simulink model "Vehicle_HIL_plant"  (R2022b)
settings: Solver=VariableStepAuto  StartTime=0.0  StopTime=inf  RelTol=1e-3
undefined symbols (not defined in the file): canChannel, MI_STATUSES
libraries: canmsglib x12, canlib x5, dspstat3 x4, simulink x2, realtime_pacer_lib x1, battery_monitor_lib x1, driver_interface_lib x1, governor_lib x1, motor_interface_lib x1, simp_vd_lib x1
settings Model: Creator=LinF  LastModifiedBy=LinF

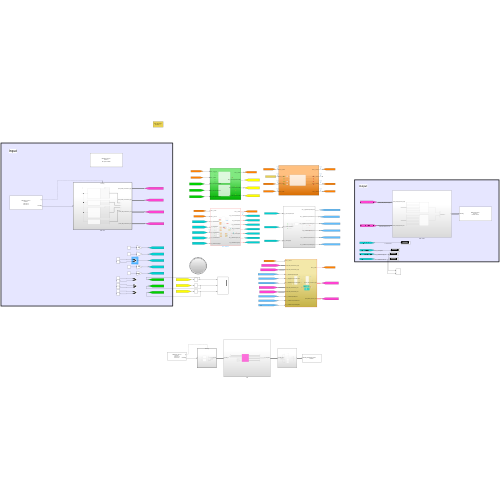
[thumbnail: Simulink's stored preview of the top-level diagram]
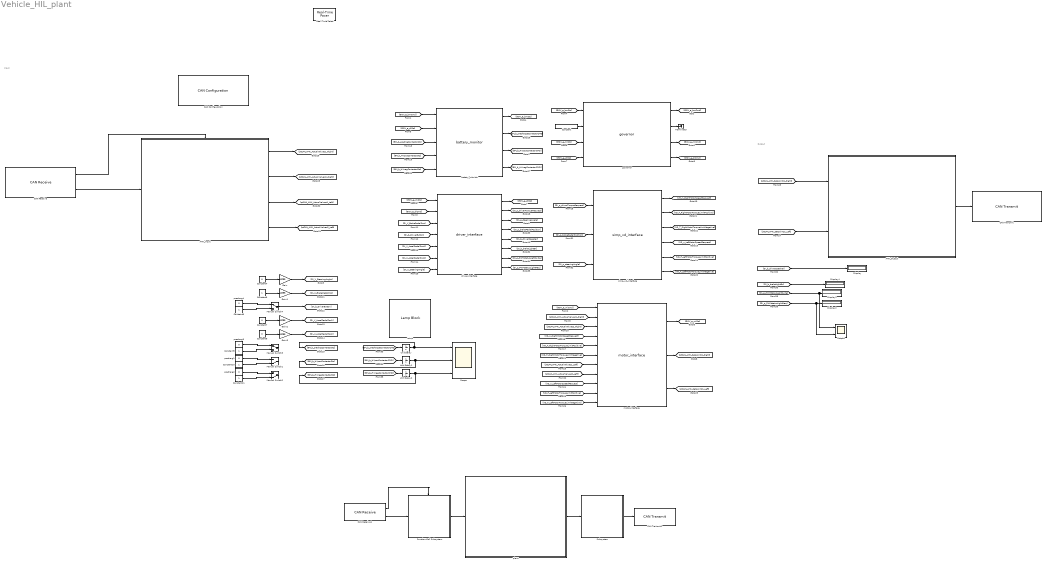
== system Vehicle_HIL_plant ==
  note: Input
  note: Output
  AMK_Input : Subsystem  TreatAsAtomicUnit=on
  AMK_Output : Subsystem
  CAN Configuration : canlib/CAN Configuration  BlockHandle=174.0005  Device=MathWorks Virtual 1 (Channel 1)  DeviceMenu=MathWorks Virtual 1 (Channel 1)  ObjConstructor=canChannel('MathWorks', 'Virtual 1', 1)  BusSpeed=500000  EnableBitParameters=off  AckMode=Normal
  CAN Receive : canlib/CAN Receive  BlockHandle=175.0005  Device=MathWorks Virtual 1 (Channel 1)  DeviceMenu=MathWorks Virtual 1 (Channel 1)  ObjConstructor=canChannel('MathWorks', 'Virtual 1', 1)  EnableStandardIDsFilter=off  StdIDsCombo=Allow all  StandardIDs=0  EnableExtendedIDsFilter=off  ExtIDsCombo=Allow all  ExtendedIDs=0  SampleTime=0.005  MsgsPerTimestep=all  InternalFilterUpdateStatus=on  BusOutput=off
  CAN Receive1 : canlib/CAN Receive  BlockHandle=178.0005  Device=MathWorks Virtual 1 (Channel 1)  DeviceMenu=MathWorks Virtual 1 (Channel 1)  ObjConstructor=canChannel('MathWorks', 'Virtual 1', 1)  EnableStandardIDsFilter=off  StdIDsCombo=Allow all  StandardIDs=0  EnableExtendedIDsFilter=off  ExtIDsCombo=Allow all  ExtendedIDs=0  SampleTime=0.005  MsgsPerTimestep=all  InternalFilterUpdateStatus=on  BusOutput=off
  CAN Transmit : canlib/CAN Transmit  BlockHandle=181.0005  Device=MathWorks Virtual 1 (Channel 1)  DeviceMenu=MathWorks Virtual 1 (Channel 1)  ObjConstructor=canChannel('MathWorks', 'Virtual 1', 1)  EnableEventTransmit=off  EnablePeriodicTransmit=on  MessagePeriod=0.005
  CAN Transmit1 : canlib/CAN Transmit  BlockHandle=183.0005  Device=MathWorks Virtual 1 (Channel 1)  DeviceMenu=MathWorks Virtual 1 (Channel 1)  ObjConstructor=canChannel('MathWorks', 'Virtual 1', 1)  EnableEventTransmit=off  EnablePeriodicTransmit=off  MessagePeriod=1.000
  Constant : Constant  Value=MI_STATUSES.STS_INIT  OutDataTypeStr=Enum: MI_STATUSES
  Constant{5..6,9..11} (5 alike) : Constant
  Constant4 : Constant  Value=0
  Constant7 : Constant  Value=0
  Constant8 : Constant  Value=0
  Display{,1..2,4} (4 alike) : Display
  Function-Call Subsystem : Subsystem  TreatAsAtomicUnit=on
  Gain{,1..3} (4 alike) : Gain  Gain=4095
  Lamp : LampBlock  LabelPosition=Hide
  Manual Switch1 : ManualSwitch  CurrentSetting=0
  Manual Switch2 : ManualSwitch  CurrentSetting=0
  Manual Switch3 : ManualSwitch
  Manual Switch4 : ManualSwitch
  Real-Time Pacer : realtime_pacer_lib/Real-Time Pacer  simTimePerRealTime=1
  Scope : Scope  NumInputPorts=3
  Scope1 : Scope  NumInputPorts=2
  Subsystem : Subsystem
  Terminator : Terminator
  Unit Delay : UnitDelay  SampleTime=-1  HasFrameUpgradeWarning=on
  Unit Delay1 : UnitDelay  SampleTime=-1  HasFrameUpgradeWarning=on
  Unit Delay2 : UnitDelay  SampleTime=-1  HasFrameUpgradeWarning=on
  battery_monitor : battery_monitor_lib/battery_monitor  SystemSampleTime=-1  VariantActivationTime=update diagram  Latency=0  AutoFrameSizeCalculation=off
  driver_interface : driver_interface_lib/driver_interface  SystemSampleTime=-1  VariantActivationTime=update diagram  Latency=0  AutoFrameSizeCalculation=off
  governor : governor_lib/governor  SystemSampleTime=-1  VariantActivationTime=update diagram  Latency=0  AutoFrameSizeCalculation=off
  motor_interface : motor_interface_lib/motor_interface  SystemSampleTime=-1  VariantActivationTime=update diagram  Latency=0  AutoFrameSizeCalculation=off
  plant : Subsystem
      settings: LibrarySourceBlock=plant_lib/plant
  precharg{1..4} (4 alike) : Constant  Value=0
  simp_vd_interface : simp_vd_lib/simp_vd_interface  SystemSampleTime=-1  VariantActivationTime=update diagram  Latency=0  AutoFrameSizeCalculation=off
  wires:
  Function-Call Subsystem/1(pt_CAN_IN) -> plant/1(pt_CAN_IN)
  CAN Receive1/2 -> Function-Call Subsystem/1(In1)
  CAN Receive1/1 -> Function-Call Subsystem/Trigger
  plant/1(pt_CAN_OUT) -> Subsystem/1(pt_CAN_OUT)
  Subsystem/1(Out1) -> CAN Transmit1/1
  Gain3/1 -> [DI_V_AccelPedalPos2]
  [DI_b_driverSpeaker] -> Display/1  "DI_b_driverSpeaker"
  Constant4/1 -> Gain/1
  Gain2/1 -> [DI_V_AccelPedalPos1]
  Manual Switch4/1 -> [DI_b_DriverButton]
  Gain1/1 -> [DI_V_BrakePedalPos]
  motor_interface/1 -> [GOV_e_miSts]
  [ptCAN_AMK_Setpoints1_Right] -> AMK_Output/1(ptCAN_AMK_Setpoints1_Right)  "ptCAN_AMK_Setpoints1_Right"
  Constant5/1 -> Gain1/1
  [VD_T_RightMotorTorqueLimitPositive] -> motor_interface/5
  [GOV_e_bmSts] -> governor/1
  AMK_Input/2(ptCAN_AMK_ActualValues2_Right) -> [ptCAN_AMK_ActualValues2_Right]
  CAN Receive/1 -> AMK_Input/Trigger
  AMK_Output/1(Out1) -> CAN Transmit/1
  AMK_Input/4(ptCAN_AMK_ActualValues2_Left) -> [ptCAN_AMK_ActualValues2_Left]
  AMK_Input/3(ptCAN_AMK_ActualValues1_Left) -> [ptCAN_AMK_ActualValues1_Left]
  CAN Receive/2 -> AMK_Input/1(In1)
  motor_interface/3 -> [ptCAN_AMK_Setpoints1_Left]
  governor/1 -> [GOV_e_bmCmd]
  governor/2 -> Terminator/1
  governor/4 -> [GOV_e_diCmd]
  motor_interface/2 -> [ptCAN_AMK_Setpoints1_Right]
  [GOV_e_diSts] -> governor/4
  [VD_T_LeftMotorTorqueLimitPositive] -> motor_interface/10
  [VD_T_RightMotorTorqueLimitNegative] -> motor_interface/6
  [VD_n_RightMotorSpeedRequest] -> motor_interface/4
  [GOV_e_miCmd] -> motor_interface/1
  [VD_T_LeftMotorTorqueLimitNegative] -> motor_interface/11
  [VD_n_LeftMotorSpeedRequest] -> motor_interface/9
  AMK_Input/1(ptCAN_AMK_ActualValues1_Right) -> [ptCAN_AMK_ActualValues1_Right]
  [ptCAN_AMK_ActualValues2_Left] -> motor_interface/8
  Constant/1 -> governor/2
  governor/3 -> [GOV_e_miCmd]
  [ptCAN_AMK_ActualValues1_Right] -> motor_interface/2
  [ptCAN_AMK_ActualValues2_Right] -> motor_interface/3
  [ptCAN_AMK_ActualValues1_Left] -> motor_interface/7
  [ptCAN_AMK_Setpoints1_Left] -> AMK_Output/2(ptCAN_AMK_Setpoints1_Left)  "ptCAN_AMK_Setpoints1_Left"
  Gain/1 -> [DI_V_SteeringAngle]
  Constant8/1 -> Gain3/1
  [GOV_e_miSts] -> governor/3
  Constant7/1 -> Gain2/1
  Constant10/1 -> Manual Switch1/2
  precharg1/1 -> Manual Switch1/1
  [BM_b_HVposContactorCMD] -> Unit Delay1/1
  precharg2/1 -> Manual Switch2/1
  Constant11/1 -> Manual Switch2/2
  [BM_b_HVnegContactorCMD] -> Unit Delay2/1
  precharg3/1 -> Manual Switch3/1
  Constant9/1 -> Manual Switch3/2
  [BM_b_prechargeContactorCMD] -> Unit Delay/1
  precharg4/1 -> Manual Switch4/1
  Constant6/1 -> Manual Switch4/2
  [BM_b_HVnegContactorSts] -> battery_monitor/5
  [GOV_e_bmCmd] -> battery_monitor/1
  battery_monitor/1 -> [GOV_e_bmSts]
  battery_monitor/2 -> [BM_b_prechargeContactorCMD]
  battery_monitor/3 -> [BM_b_HVposContactorCMD]
  [BM_b_prechrgContactorSts] -> battery_monitor/3
  battery_monitor/4 -> [BM_b_HVnegContactorCMD]
  [BM_b_HVposContactorSts] -> battery_monitor/4
  [GOV_e_diSts] -> battery_monitor/2
  Unit Delay/1 -> [BM_b_prechrgContactorSts], Scope/1
  Unit Delay1/1 -> [BM_b_HVposContactorSts], Scope/2
  Unit Delay2/1 -> [BM_b_HVnegContactorSts], Scope/3
  [DI_b_brakeLightEn] -> Display4/1  "DI_b_brakeLightEn"
  driver_interface/8 -> [DI_p_PWMstatusLightFreq]
  [GOV_e_miSts] -> driver_interface/1
  [GOV_e_diCmd] -> driver_interface/2
  [DI_V_AccelPedalPos1] -> driver_interface/5
  [DI_V_AccelPedalPos2] -> driver_interface/6
  driver_interface/6 -> [DI_b_brakeLightEn]
  [DI_b_DriverButton] -> driver_interface/4
  [DI_V_BrakePedalPos] -> driver_interface/3
  driver_interface/2 -> [DI_p_driverTorqueRequest]
  driver_interface/5 -> [DI_b_driverSpeaker]
  driver_interface/1 -> [GOV_e_diSts]
  driver_interface/4 -> [DI_p_brakePedalPosition]
  [DI_V_SteeringAngle] -> driver_interface/7
  driver_interface/3 -> [DI_p_steeringAngle]
  driver_interface/7 -> [DI_p_PWMstatusLightCycle]
  [DI_p_PWMstatusLightFreq] -> Scope1/2, Display2/1  "DI_p_PWMstatusLightFreq"
  [DI_p_PWMstatusLightCycle] -> Scope1/1, Display1/1  "DI_p_PWMstatusLightCycle"
  simp_vd_interface/4 -> [VD_n_LeftMotorSpeedRequest]
  simp_vd_interface/2 -> [VD_T_RightMotorTorqueLimitPositive]
  [DI_p_driverTorqueRequest] -> simp_vd_interface/1
  simp_vd_interface/6 -> [VD_T_LeftMotorTorqueLimitNegative]
  simp_vd_interface/3 -> [VD_T_RightMotorTorqueLimitNegative]
  [DI_p_steeringAngle] -> simp_vd_interface/3
  [DI_p_brakePedalPosition] -> simp_vd_interface/2
  simp_vd_interface/5 -> [VD_T_LeftMotorTorqueLimitPositive]
  simp_vd_interface/1 -> [VD_n_RightMotorSpeedRequest]

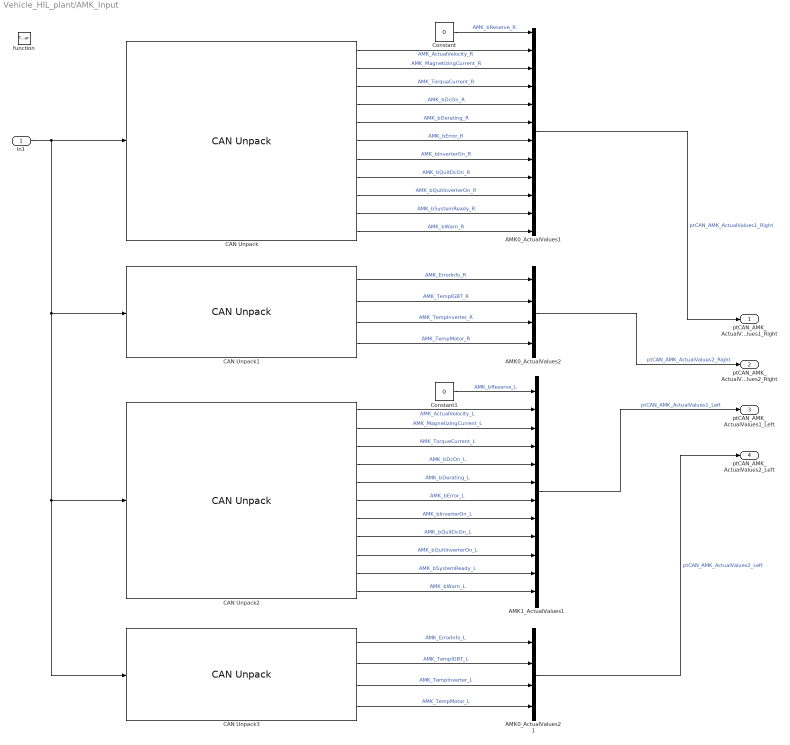
== system Vehicle_HIL_plant/AMK_Input ==
  In1 : Inport
  function : TriggerPort  TriggerType=function-call  VariantControl=(inherit)
  "AMK0_ActualValues1 " : BusCreator  Inputs=12
  "AMK0_ActualValues2 " : BusCreator  Inputs=4
  AMK0_ActualValues2 1 : BusCreator  Inputs=4
  AMK1_ActualValues1 : BusCreator  Inputs=12
  CAN Unpack : canmsglib/CAN Unpack  CANdbFile=C:\Users\LinF\Documents\MACFE\Embedded\CAN_Stuff\CAN_Databases\CAN_AMKInverter.dbc  MsgList=AMK1_ActualValues1  MsgName=AMK1_ActualValues1  MsgIDType=Standard (11-bit identifier)  MsgIdentifier=645  MsgLength=8  SignalInfo={'AMK_ActualVelocity','16','16','LE','signed','Standard','0','1','0','-Inf','Inf';'AMK_MagnetizingCurrent','48','16','LE','signed','Standard','0','1','0','-Inf','Inf';'AMK_TorqueCurrent','32','16','LE','signed','Standard','0','1','0','-Inf','Inf';'AMK_bDcOn','12','1','LE','unsigned','Standard','0','1','0','-Inf','Inf';'AMK_bDerating','15','1','LE','unsigned','Standard','0','1','0','-Inf','Inf';'AMK_bError','9','1','LE','unsigned','Standard','0','1','0','-Inf','Inf';'AMK_bInverterOn','14','1','LE','unsigned','Standard','0','1','0','-Inf','Inf';'AMK_bQuitDcOn','11','1','LE','unsigned','Standard','0','1','0','-Inf','Inf';'AMK_bQuitInverterOn','13','1','LE','unsigned','Standard','0','1','0','-Inf','Inf';'AMK_bSystemReady','8','1','LE','unsigned','Standard','0','1','0','-Inf','Inf';'AMK_bWarn','10','1','LE','unsigned','Standard','0','1','0','-Inf','Inf'}  IDPort=off  TimestampPort=off  ErrorPort=off  RemotePort=off  LengthPort=off  StatusPort=off  ApplyMinMax=off
      settings: LibrarySourceBlock=canlib/CAN Unpack  DataFormat=CANdb specified signals
  CAN Unpack1 : canmsglib/CAN Unpack  CANdbFile=C:\Users\LinF\Documents\MACFE\Embedded\CAN_Stuff\CAN_Databases\CAN_AMKInverter.dbc  MsgList=AMK1_ActualValues2  MsgName=AMK1_ActualValues2  MsgIDType=Standard (11-bit identifier)  MsgIdentifier=647  MsgLength=8  SignalInfo={'AMK_ErrorInfo','32','16','LE','unsigned','Standard','0','1','0','0','65535';'AMK_TempIGBT','48','16','LE','signed','Standard','0','0.1','0','-3276.8','3276.7';'AMK_TempInverter','16','16','LE','signed','Standard','0','0.1','0','-3276.8','3276.7';'AMK_TempMotor','0','16','LE','signed','Standard','0','0.1','0','-3276.8','3276.7'}  IDPort=off  TimestampPort=off  ErrorPort=off  RemotePort=off  LengthPort=off  StatusPort=off  ApplyMinMax=off
      settings: LibrarySourceBlock=canlib/CAN Unpack  DataFormat=CANdb specified signals
  CAN Unpack2 : canmsglib/CAN Unpack  CANdbFile=C:\Users\LinF\Documents\MACFE\Embedded\CAN_Stuff\CAN_Databases\CAN_AMKInverter.dbc  MsgList=AMK0_ActualValues1  MsgName=AMK0_ActualValues1  MsgIDType=Standard (11-bit identifier)  MsgIdentifier=644  MsgLength=8  SignalInfo={'AMK_ActualVelocity','16','16','LE','signed','Standard','0','1','0','-Inf','Inf';'AMK_MagnetizingCurrent','48','16','LE','signed','Standard','0','1','0','-Inf','Inf';'AMK_TorqueCurrent','32','16','LE','signed','Standard','0','1','0','-Inf','Inf';'AMK_bDcOn','12','1','LE','unsigned','Standard','0','1','0','-Inf','Inf';'AMK_bDerating','15','1','LE','unsigned','Standard','0','1','0','-Inf','Inf';'AMK_bError','9','1','LE','unsigned','Standard','0','1','0','-Inf','Inf';'AMK_bInverterOn','14','1','LE','unsigned','Standard','0','1','0','-Inf','Inf';'AMK_bQuitDcOn','11','1','LE','unsigned','Standard','0','1','0','-Inf','Inf';'AMK_bQuitInverterOn','13','1','LE','unsigned','Standard','0','1','0','-Inf','Inf';'AMK_bSystemReady','8','1','LE','unsigned','Standard','0','1','0','-Inf','Inf';'AMK_bWarn','10','1','LE','unsigned','Standard','0','1','0','-Inf','Inf'}  IDPort=off  TimestampPort=off  ErrorPort=off  RemotePort=off  LengthPort=off  StatusPort=off  ApplyMinMax=off
      settings: LibrarySourceBlock=canlib/CAN Unpack  DataFormat=CANdb specified signals
  CAN Unpack3 : canmsglib/CAN Unpack  CANdbFile=C:\Users\LinF\Documents\MACFE\Embedded\CAN_Stuff\CAN_Databases\CAN_AMKInverter.dbc  MsgList=AMK0_ActualValues2  MsgName=AMK0_ActualValues2  MsgIDType=Standard (11-bit identifier)  MsgIdentifier=646  MsgLength=8  SignalInfo={'AMK_ErrorInfo','32','16','LE','unsigned','Standard','0','1','0','0','65535';'AMK_TempIGBT','48','16','LE','signed','Standard','0','0.1','0','-3276.8','3276.7';'AMK_TempInverter','16','16','LE','signed','Standard','0','0.1','0','-3276.8','3276.7';'AMK_TempMotor','0','16','LE','signed','Standard','0','0.1','0','-3276.8','3276.7'}  IDPort=off  TimestampPort=off  ErrorPort=off  RemotePort=off  LengthPort=off  StatusPort=off  ApplyMinMax=off
      settings: LibrarySourceBlock=canlib/CAN Unpack  DataFormat=CANdb specified signals
  Constant : Constant  Value=0
  Constant1 : Constant  Value=0
  ptCAN_AMK_ActualValues1_Right : Outport
  ptCAN_AMK_ActualValues2_Right : Outport  Port=2
  ptCAN_AMK_ActualValues1_Left : Outport  Port=3
  ptCAN_AMK_ActualValues2_Left : Outport  Port=4
  wires:
  In1/1 -> CAN Unpack3/1, CAN Unpack2/1, CAN Unpack1/1, CAN Unpack/1
  CAN Unpack/1 -> "AMK0_ActualValues1 "/2  "AMK_ActualVelocity_R"
  CAN Unpack/2 -> "AMK0_ActualValues1 "/3  "AMK_MagnetizingCurrent_R"
  CAN Unpack/3 -> "AMK0_ActualValues1 "/4  "AMK_TorqueCurrent_R"
  CAN Unpack/4 -> "AMK0_ActualValues1 "/5  "AMK_bDcOn_R"
  CAN Unpack/5 -> "AMK0_ActualValues1 "/6  "AMK_bDerating_R"
  CAN Unpack/6 -> "AMK0_ActualValues1 "/7  "AMK_bError_R"
  CAN Unpack/7 -> "AMK0_ActualValues1 "/8  "AMK_bInverterOn_R"
  CAN Unpack/8 -> "AMK0_ActualValues1 "/9  "AMK_bQuitDcOn_R"
  CAN Unpack/9 -> "AMK0_ActualValues1 "/10  "AMK_bQuitInverterOn_R"
  CAN Unpack/10 -> "AMK0_ActualValues1 "/11  "AMK_bSystemReady_R"
  CAN Unpack/11 -> "AMK0_ActualValues1 "/12  "AMK_bWarn_R"
  "AMK0_ActualValues1 "/1 -> ptCAN_AMK_ActualValues1_Right/1  "ptCAN_AMK_ActualValues1_Right"
  CAN Unpack2/1 -> AMK1_ActualValues1/2  "AMK_ActualVelocity_L"
  CAN Unpack2/10 -> AMK1_ActualValues1/11  "AMK_bSystemReady_L"
  CAN Unpack2/6 -> AMK1_ActualValues1/7  "AMK_bError_L"
  CAN Unpack2/9 -> AMK1_ActualValues1/10  "AMK_bQuitInverterOn_L"
  CAN Unpack2/2 -> AMK1_ActualValues1/3  "AMK_MagnetizingCurrent_L"
  CAN Unpack2/3 -> AMK1_ActualValues1/4  "AMK_TorqueCurrent_L"
  AMK1_ActualValues1/1 -> ptCAN_AMK_ActualValues1_Left/1  "ptCAN_AMK_ActualValues1_Left"
  CAN Unpack2/8 -> AMK1_ActualValues1/9  "AMK_bQuitDcOn_L"
  CAN Unpack2/4 -> AMK1_ActualValues1/5  "AMK_bDcOn_L"
  CAN Unpack2/5 -> AMK1_ActualValues1/6  "AMK_bDerating_L"
  CAN Unpack2/11 -> AMK1_ActualValues1/12  "AMK_bWarn_L"
  CAN Unpack2/7 -> AMK1_ActualValues1/8  "AMK_bInverterOn_L"
  CAN Unpack1/1 -> "AMK0_ActualValues2 "/1  "AMK_ErrorInfo_R"
  CAN Unpack1/2 -> "AMK0_ActualValues2 "/2  "AMK_TempIGBT_R"
  CAN Unpack1/3 -> "AMK0_ActualValues2 "/3  "AMK_TempInverter_R"
  CAN Unpack1/4 -> "AMK0_ActualValues2 "/4  "AMK_TempMotor_R"
  "AMK0_ActualValues2 "/1 -> ptCAN_AMK_ActualValues2_Right/1  "ptCAN_AMK_ActualValues2_Right"
  CAN Unpack3/1 -> AMK0_ActualValues2 1/1  "AMK_ErrorInfo_L"
  CAN Unpack3/4 -> AMK0_ActualValues2 1/4  "AMK_TempMotor_L"
  AMK0_ActualValues2 1/1 -> ptCAN_AMK_ActualValues2_Left/1  "ptCAN_AMK_ActualValues2_Left"
  CAN Unpack3/3 -> AMK0_ActualValues2 1/3  "AMK_TempInverter_L"
  CAN Unpack3/2 -> AMK0_ActualValues2 1/2  "AMK_TempIGBT_L"
  Constant/1 -> "AMK0_ActualValues1 "/1  "AMK_bReserve_R"
  Constant1/1 -> AMK1_ActualValues1/1  "AMK_bReserve_L"

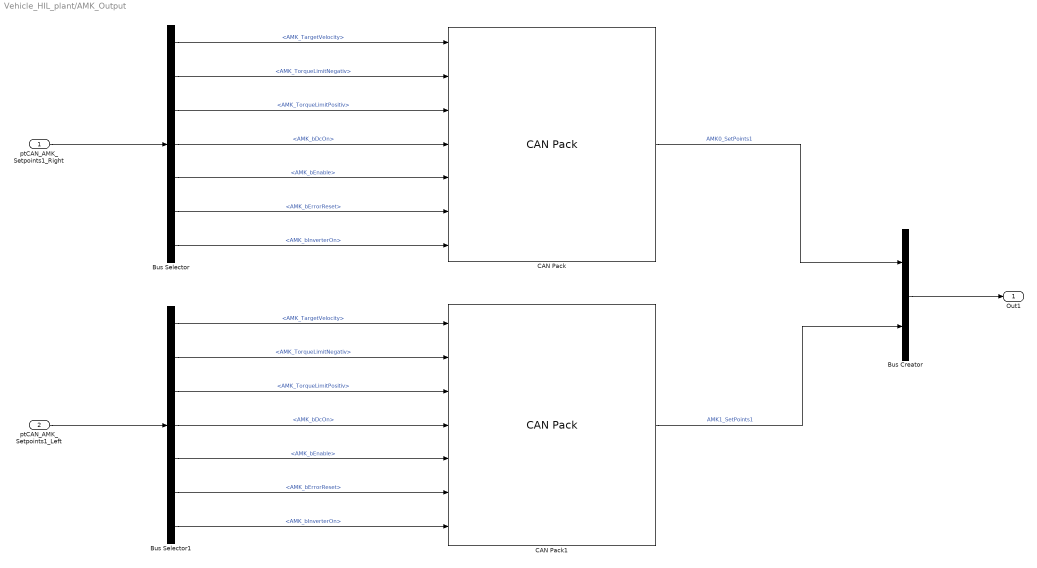
== system Vehicle_HIL_plant/AMK_Output ==
  ptCAN_AMK_Setpoints1_Right : Inport
  ptCAN_AMK_Setpoints1_Left : Inport  Port=2
  Bus Creator : BusCreator  Inputs=2
  Bus Selector : BusSelector  OutputSignals=AMK_TargetVelocity,AMK_TorqueLimitNegativ,AMK_TorqueLimitPositiv,AMK_bDcOn,AMK_bEnable,AMK_bErrorReset,AMK_bInverterOn
  Bus Selector1 : BusSelector  OutputSignals=AMK_TargetVelocity,AMK_TorqueLimitNegativ,AMK_TorqueLimitPositiv,AMK_bDcOn,AMK_bEnable,AMK_bErrorReset,AMK_bInverterOn
  CAN Pack : canmsglib/CAN Pack  CANdbFile=C:\Users\LinF\Documents\MACFE\Embedded\CAN_Stuff\CAN_Databases\CAN_AMKInverter.dbc  MsgList=AMK1_SetPoints1  MsgName=AMK1_SetPoints1  MsgIDType=Standard (11-bit identifier)  MsgIdentifier=390  MsgLength=8  Remote=off  ApplyMinMax=off  BusOutput=off  SignalInfo={'AMK_TargetVelocity','16','16','LE','signed','Standard','0','1','0','-Inf','Inf';'AMK_TorqueLimitNegativ','48','16','LE','signed','Standard','0','1','0','-Inf','Inf';'AMK_TorqueLimitPositiv','32','16','LE','signed','Standard','0','1','0','-Inf','Inf';'AMK_bDcOn','9','1','LE','unsigned','Standard','0','1','0','-Inf','Inf';'AMK_bEnable','10','1','LE','unsigned','Standard','0','1','0','-Inf','Inf';'AMK_bErrorReset','11','1','LE','unsigned','Standard','0','1','0','-Inf','Inf';'AMK_bInverterOn','8','1','LE','unsigned','Standard','0','1','0','-Inf','Inf'}
      settings: LibrarySourceBlock=canlib/CAN Pack  DataFormat=CANdb specified signals
  CAN Pack1 : canmsglib/CAN Pack  CANdbFile=C:\Users\LinF\Documents\MACFE\Embedded\CAN_Stuff\CAN_Databases\CAN_AMKInverter.dbc  MsgList=AMK0_SetPoints1  MsgName=AMK0_SetPoints1  MsgIDType=Standard (11-bit identifier)  MsgIdentifier=389  MsgLength=8  Remote=off  ApplyMinMax=off  BusOutput=off  SignalInfo={'AMK_TargetVelocity','16','16','LE','signed','Standard','0','1','0','-Inf','Inf';'AMK_TorqueLimitNegativ','48','16','LE','signed','Standard','0','1','0','-Inf','Inf';'AMK_TorqueLimitPositiv','32','16','LE','signed','Standard','0','1','0','-Inf','Inf';'AMK_bDcOn','9','1','LE','unsigned','Standard','0','1','0','-Inf','Inf';'AMK_bEnable','10','1','LE','unsigned','Standard','0','1','0','-Inf','Inf';'AMK_bErrorReset','11','1','LE','unsigned','Standard','0','1','0','-Inf','Inf';'AMK_bInverterOn','8','1','LE','unsigned','Standard','0','1','0','-Inf','Inf'}
      settings: LibrarySourceBlock=canlib/CAN Pack  DataFormat=CANdb specified signals
  Out1 : Outport
  wires:
  CAN Pack/1 -> Bus Creator/1  "AMK0_SetPoints1"
  CAN Pack1/1 -> Bus Creator/2  "AMK1_SetPoints1"
  Bus Selector/7 -> CAN Pack/7  "<AMK_bInverterOn>"
  Bus Selector/4 -> CAN Pack/4  "<AMK_bDcOn>"
  Bus Selector/5 -> CAN Pack/5  "<AMK_bEnable>"
  Bus Selector/6 -> CAN Pack/6  "<AMK_bErrorReset>"
  Bus Selector/1 -> CAN Pack/1  "<AMK_TargetVelocity>"
  Bus Selector/3 -> CAN Pack/3  "<AMK_TorqueLimitPositiv>"
  Bus Selector/2 -> CAN Pack/2  "<AMK_TorqueLimitNegativ>"
  Bus Creator/1 -> Out1/1
  Bus Selector1/1 -> CAN Pack1/1  "<AMK_TargetVelocity>"
  Bus Selector1/3 -> CAN Pack1/3  "<AMK_TorqueLimitPositiv>"
  Bus Selector1/2 -> CAN Pack1/2  "<AMK_TorqueLimitNegativ>"
  Bus Selector1/4 -> CAN Pack1/4  "<AMK_bDcOn>"
  Bus Selector1/5 -> CAN Pack1/5  "<AMK_bEnable>"
  Bus Selector1/6 -> CAN Pack1/6  "<AMK_bErrorReset>"
  Bus Selector1/7 -> CAN Pack1/7  "<AMK_bInverterOn>"
  ptCAN_AMK_Setpoints1_Right/1 -> Bus Selector/1
  ptCAN_AMK_Setpoints1_Left/1 -> Bus Selector1/1

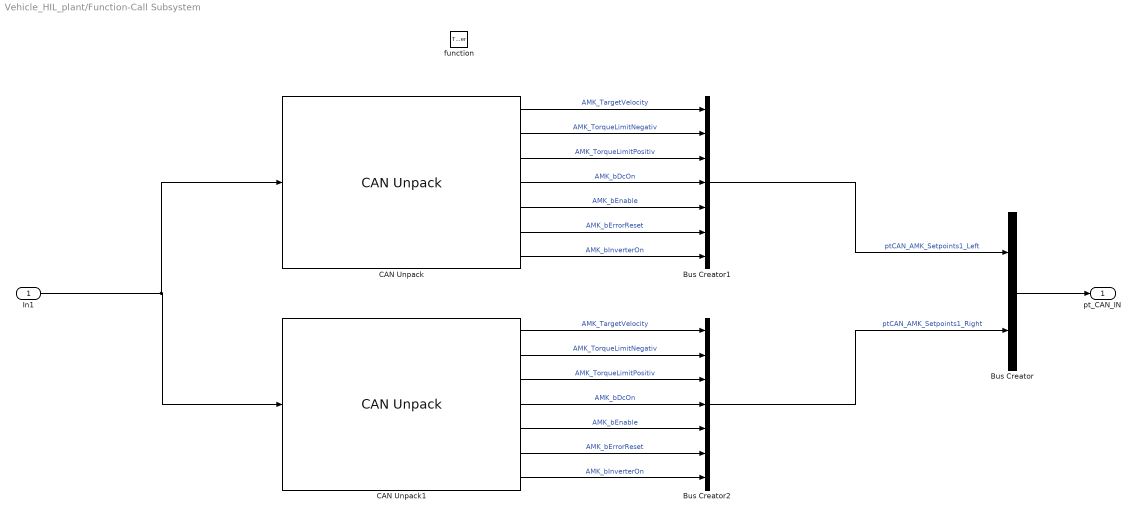
== system Vehicle_HIL_plant/Function-Call Subsystem ==
  In1 : Inport
  function : TriggerPort  TriggerType=function-call  VariantControl=(inherit)
  Bus Creator : BusCreator  Inputs=2
  Bus Creator1 : BusCreator  Inputs=7
  Bus Creator2 : BusCreator  Inputs=7
  CAN Unpack : canmsglib/CAN Unpack  CANdbFile=C:\Users\LinF\Documents\MACFE\Embedded\CAN_Stuff\CAN_Databases\CAN_AMKInverter.dbc  MsgList=AMK0_SetPoints1  MsgName=AMK0_SetPoints1  MsgIDType=Standard (11-bit identifier)  MsgIdentifier=389  MsgLength=8  SignalInfo={'AMK_TargetVelocity','16','16','LE','signed','Standard','0','1','0','-Inf','Inf';'AMK_TorqueLimitNegativ','48','16','LE','signed','Standard','0','1','0','-Inf','Inf';'AMK_TorqueLimitPositiv','32','16','LE','signed','Standard','0','1','0','-Inf','Inf';'AMK_bDcOn','9','1','LE','unsigned','Standard','0','1','0','-Inf','Inf';'AMK_bEnable','10','1','LE','unsigned','Standard','0','1','0','-Inf','Inf';'AMK_bErrorReset','11','1','LE','unsigned','Standard','0','1','0','-Inf','Inf';'AMK_bInverterOn','8','1','LE','unsigned','Standard','0','1','0','-Inf','Inf'}  IDPort=off  TimestampPort=off  ErrorPort=off  RemotePort=off  LengthPort=off  StatusPort=off  ApplyMinMax=off
      settings: LibrarySourceBlock=canlib/CAN Unpack  DataFormat=CANdb specified signals
  CAN Unpack1 : canmsglib/CAN Unpack  CANdbFile=C:\Users\LinF\Documents\MACFE\Embedded\CAN_Stuff\CAN_Databases\CAN_AMKInverter.dbc  MsgList=AMK1_SetPoints1  MsgName=AMK1_SetPoints1  MsgIDType=Standard (11-bit identifier)  MsgIdentifier=390  MsgLength=8  SignalInfo={'AMK_TargetVelocity','16','16','LE','signed','Standard','0','1','0','-Inf','Inf';'AMK_TorqueLimitNegativ','48','16','LE','signed','Standard','0','1','0','-Inf','Inf';'AMK_TorqueLimitPositiv','32','16','LE','signed','Standard','0','1','0','-Inf','Inf';'AMK_bDcOn','9','1','LE','unsigned','Standard','0','1','0','-Inf','Inf';'AMK_bEnable','10','1','LE','unsigned','Standard','0','1','0','-Inf','Inf';'AMK_bErrorReset','11','1','LE','unsigned','Standard','0','1','0','-Inf','Inf';'AMK_bInverterOn','8','1','LE','unsigned','Standard','0','1','0','-Inf','Inf'}  IDPort=off  TimestampPort=off  ErrorPort=off  RemotePort=off  LengthPort=off  StatusPort=off  ApplyMinMax=off
      settings: LibrarySourceBlock=canlib/CAN Unpack  DataFormat=CANdb specified signals
  pt_CAN_IN : Outport
  wires:
  Bus Creator/1 -> pt_CAN_IN/1
  Bus Creator2/1 -> Bus Creator/2  "ptCAN_AMK_Setpoints1_Right"
  Bus Creator1/1 -> Bus Creator/1  "ptCAN_AMK_Setpoints1_Left"
  In1/1 -> CAN Unpack/1, CAN Unpack1/1
  CAN Unpack/1 -> Bus Creator1/1  "AMK_TargetVelocity"
  CAN Unpack/2 -> Bus Creator1/2  "AMK_TorqueLimitNegativ"
  CAN Unpack/3 -> Bus Creator1/3  "AMK_TorqueLimitPositiv"
  CAN Unpack/4 -> Bus Creator1/4  "AMK_bDcOn"
  CAN Unpack/5 -> Bus Creator1/5  "AMK_bEnable"
  CAN Unpack/6 -> Bus Creator1/6  "AMK_bErrorReset"
  CAN Unpack/7 -> Bus Creator1/7  "AMK_bInverterOn"
  CAN Unpack1/3 -> Bus Creator2/3  "AMK_TorqueLimitPositiv"
  CAN Unpack1/6 -> Bus Creator2/6  "AMK_bErrorReset"
  CAN Unpack1/4 -> Bus Creator2/4  "AMK_bDcOn"
  CAN Unpack1/7 -> Bus Creator2/7  "AMK_bInverterOn"
  CAN Unpack1/2 -> Bus Creator2/2  "AMK_TorqueLimitNegativ"
  CAN Unpack1/5 -> Bus Creator2/5  "AMK_bEnable"
  CAN Unpack1/1 -> Bus Creator2/1  "AMK_TargetVelocity"

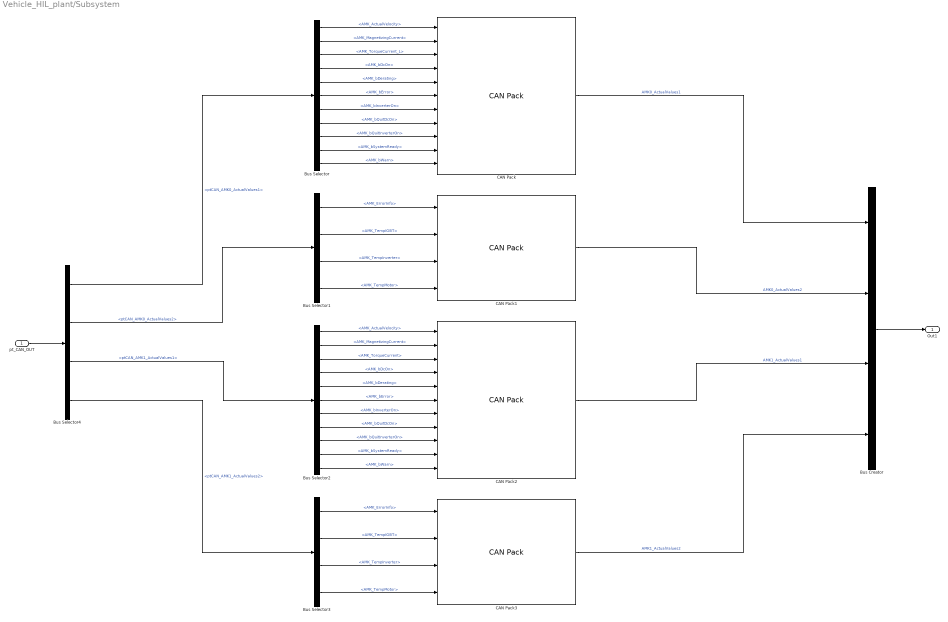
== system Vehicle_HIL_plant/Subsystem ==
  pt_CAN_OUT : Inport
  Bus Creator : BusCreator  Inputs=4
  Bus Selector : BusSelector  OutputSignals=AMK_ActualVelocity,AMK_MagnetizingCurrent,AMK_TorqueCurrent_L,AMK_bDcOn,AMK_bDerating,AMK_bError,AMK_bInverterOn,AMK_bQuitDcOn,AMK_bQuitInverterOn,AMK_bSystemReady,AMK_bWarn
  Bus Selector1 : BusSelector  OutputSignals=AMK_ErrorInfo,AMK_TempIGBT,AMK_TempInverter,AMK_TempMotor
  Bus Selector2 : BusSelector  OutputSignals=AMK_ActualVelocity,AMK_MagnetizingCurrent,AMK_TorqueCurrent,AMK_bDcOn,AMK_bDerating,AMK_bError,AMK_bInverterOn,AMK_bQuitDcOn,AMK_bQuitInverterOn,AMK_bSystemReady,AMK_bWarn
  Bus Selector3 : BusSelector  OutputSignals=AMK_ErrorInfo,AMK_TempIGBT,AMK_TempInverter,AMK_TempMotor
  Bus Selector4 : BusSelector  OutputSignals=ptCAN_AMK0_ActualValues1,ptCAN_AMK0_ActualValues2,ptCAN_AMK1_ActualValues1,ptCAN_AMK1_ActualValues2
  CAN Pack : canmsglib/CAN Pack  CANdbFile=C:\Users\LinF\Documents\MACFE\Embedded\CAN_Stuff\CAN_Databases\CAN_AMKInverter.dbc  MsgList=AMK0_ActualValues1  MsgName=AMK0_ActualValues1  MsgIDType=Standard (11-bit identifier)  MsgIdentifier=644  MsgLength=8  Remote=off  ApplyMinMax=off  BusOutput=off  SignalInfo={'AMK_ActualVelocity','16','16','LE','signed','Standard','0','1','0','-Inf','Inf';'AMK_MagnetizingCurrent','48','16','LE','signed','Standard','0','1','0','-Inf','Inf';'AMK_TorqueCurrent','32','16','LE','signed','Standard','0','1','0','-Inf','Inf';'AMK_bDcOn','12','1','LE','unsigned','Standard','0','1','0','-Inf','Inf';'AMK_bDerating','15','1','LE','unsigned','Standard','0','1','0','-Inf','Inf';'AMK_bError','9','1','LE','unsigned','Standard','0','1','0','-Inf','Inf';'AMK_bInverterOn','14','1','LE','unsigned','Standard','0','1','0','-Inf','Inf';'AMK_bQuitDcOn','11','1','LE','unsigned','Standard','0','1','0','-Inf','Inf';'AMK_bQuitInverterOn','13','1','LE','unsigned','Standard','0','1','0','-Inf','Inf';'AMK_bSystemReady','8','1','LE','unsigned','Standard','0','1','0','-Inf','Inf';'AMK_bWarn','10','1','LE','unsigned','Standard','0','1','0','-Inf','Inf'}
      settings: LibrarySourceBlock=canlib/CAN Pack  DataFormat=CANdb specified signals
  CAN Pack1 : canmsglib/CAN Pack  CANdbFile=C:\Users\LinF\Documents\MACFE\Embedded\CAN_Stuff\CAN_Databases\CAN_AMKInverter.dbc  MsgList=AMK0_ActualValues2  MsgName=AMK0_ActualValues2  MsgIDType=Standard (11-bit identifier)  MsgIdentifier=646  MsgLength=8  Remote=off  ApplyMinMax=off  BusOutput=off  SignalInfo={'AMK_ErrorInfo','32','16','LE','unsigned','Standard','0','1','0','0','65535';'AMK_TempIGBT','48','16','LE','signed','Standard','0','0.1','0','-3276.8','3276.7';'AMK_TempInverter','16','16','LE','signed','Standard','0','0.1','0','-3276.8','3276.7';'AMK_TempMotor','0','16','LE','signed','Standard','0','0.1','0','-3276.8','3276.7'}
      settings: LibrarySourceBlock=canlib/CAN Pack  DataFormat=CANdb specified signals
  CAN Pack2 : canmsglib/CAN Pack  CANdbFile=C:\Users\LinF\Documents\MACFE\Embedded\CAN_Stuff\CAN_Databases\CAN_AMKInverter.dbc  MsgList=AMK1_ActualValues1  MsgName=AMK1_ActualValues1  MsgIDType=Standard (11-bit identifier)  MsgIdentifier=645  MsgLength=8  Remote=off  ApplyMinMax=off  BusOutput=off  SignalInfo={'AMK_ActualVelocity','16','16','LE','signed','Standard','0','1','0','-Inf','Inf';'AMK_MagnetizingCurrent','48','16','LE','signed','Standard','0','1','0','-Inf','Inf';'AMK_TorqueCurrent','32','16','LE','signed','Standard','0','1','0','-Inf','Inf';'AMK_bDcOn','12','1','LE','unsigned','Standard','0','1','0','-Inf','Inf';'AMK_bDerating','15','1','LE','unsigned','Standard','0','1','0','-Inf','Inf';'AMK_bError','9','1','LE','unsigned','Standard','0','1','0','-Inf','Inf';'AMK_bInverterOn','14','1','LE','unsigned','Standard','0','1','0','-Inf','Inf';'AMK_bQuitDcOn','11','1','LE','unsigned','Standard','0','1','0','-Inf','Inf';'AMK_bQuitInverterOn','13','1','LE','unsigned','Standard','0','1','0','-Inf','Inf';'AMK_bSystemReady','8','1','LE','unsigned','Standard','0','1','0','-Inf','Inf';'AMK_bWarn','10','1','LE','unsigned','Standard','0','1','0','-Inf','Inf'}
      settings: LibrarySourceBlock=canlib/CAN Pack  DataFormat=CANdb specified signals
  CAN Pack3 : canmsglib/CAN Pack  CANdbFile=C:\Users\LinF\Documents\MACFE\Embedded\CAN_Stuff\CAN_Databases\CAN_AMKInverter.dbc  MsgList=AMK1_ActualValues2  MsgName=AMK1_ActualValues2  MsgIDType=Standard (11-bit identifier)  MsgIdentifier=647  MsgLength=8  Remote=off  ApplyMinMax=off  BusOutput=off  SignalInfo={'AMK_ErrorInfo','32','16','LE','unsigned','Standard','0','1','0','0','65535';'AMK_TempIGBT','48','16','LE','signed','Standard','0','0.1','0','-3276.8','3276.7';'AMK_TempInverter','16','16','LE','signed','Standard','0','0.1','0','-3276.8','3276.7';'AMK_TempMotor','0','16','LE','signed','Standard','0','0.1','0','-3276.8','3276.7'}
      settings: LibrarySourceBlock=canlib/CAN Pack  DataFormat=CANdb specified signals
  Out1 : Outport
  wires:
  CAN Pack/1 -> Bus Creator/1  "AMK0_ActualValues1"
  CAN Pack1/1 -> Bus Creator/2  "AMK0_ActualValues2"
  CAN Pack2/1 -> Bus Creator/3  "AMK1_ActualValues1"
  CAN Pack3/1 -> Bus Creator/4  "AMK1_ActualValues2"
  Bus Selector4/1 -> Bus Selector/1  "<ptCAN_AMK0_ActualValues1>"
  Bus Selector4/2 -> Bus Selector1/1  "<ptCAN_AMK0_ActualValues2>"
  Bus Selector4/3 -> Bus Selector2/1  "<ptCAN_AMK1_ActualValues1>"
  Bus Selector4/4 -> Bus Selector3/1  "<ptCAN_AMK1_ActualValues2>"
  pt_CAN_OUT/1 -> Bus Selector4/1
  Bus Creator/1 -> Out1/1
  Bus Selector/1 -> CAN Pack/1  "<AMK_ActualVelocity>"
  Bus Selector/3 -> CAN Pack/3  "<AMK_TorqueCurrent_L>"
  Bus Selector/2 -> CAN Pack/2  "<AMK_MagnetizingCurrent>"
  Bus Selector/4 -> CAN Pack/4  "<AMK_bDcOn>"
  Bus Selector/5 -> CAN Pack/5  "<AMK_bDerating>"
  Bus Selector/6 -> CAN Pack/6  "<AMK_bError>"
  Bus Selector/7 -> CAN Pack/7  "<AMK_bInverterOn>"
  Bus Selector/8 -> CAN Pack/8  "<AMK_bQuitDcOn>"
  Bus Selector/9 -> CAN Pack/9  "<AMK_bQuitInverterOn>"
  Bus Selector/10 -> CAN Pack/10  "<AMK_bSystemReady>"
  Bus Selector/11 -> CAN Pack/11  "<AMK_bWarn>"
  Bus Selector1/1 -> CAN Pack1/1  "<AMK_ErrorInfo>"
  Bus Selector1/2 -> CAN Pack1/2  "<AMK_TempIGBT>"
  Bus Selector1/3 -> CAN Pack1/3  "<AMK_TempInverter>"
  Bus Selector1/4 -> CAN Pack1/4  "<AMK_TempMotor>"
  Bus Selector2/3 -> CAN Pack2/3  "<AMK_TorqueCurrent>"
  Bus Selector3/1 -> CAN Pack3/1  "<AMK_ErrorInfo>"
  Bus Selector2/7 -> CAN Pack2/7  "<AMK_bInverterOn>"
  Bus Selector2/4 -> CAN Pack2/4  "<AMK_bDcOn>"
  Bus Selector2/2 -> CAN Pack2/2  "<AMK_MagnetizingCurrent>"
  Bus Selector3/4 -> CAN Pack3/4  "<AMK_TempMotor>"
  Bus Selector3/2 -> CAN Pack3/2  "<AMK_TempIGBT>"
  Bus Selector2/5 -> CAN Pack2/5  "<AMK_bDerating>"
  Bus Selector2/10 -> CAN Pack2/10  "<AMK_bSystemReady>"
  Bus Selector3/3 -> CAN Pack3/3  "<AMK_TempInverter>"
  Bus Selector2/8 -> CAN Pack2/8  "<AMK_bQuitDcOn>"
  Bus Selector2/6 -> CAN Pack2/6  "<AMK_bError>"
  Bus Selector2/11 -> CAN Pack2/11  "<AMK_bWarn>"
  Bus Selector2/1 -> CAN Pack2/1  "<AMK_ActualVelocity>"
  Bus Selector2/9 -> CAN Pack2/9  "<AMK_bQuitInverterOn>"

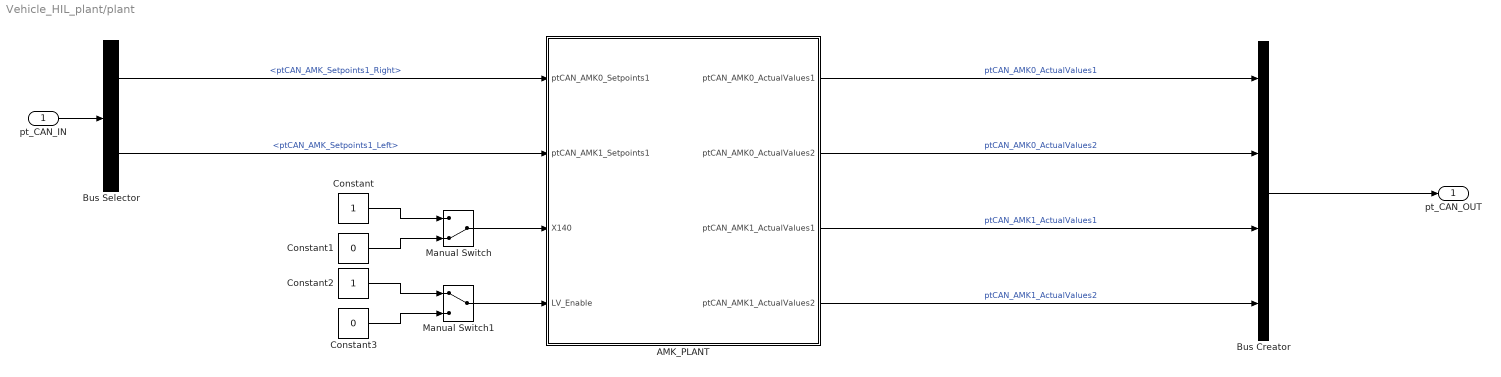
== system Vehicle_HIL_plant/plant ==
  pt_CAN_IN : Inport
  AMK_PLANT : Subsystem
  Bus Creator : BusCreator  Inputs=4
  Bus Selector : BusSelector  OutputSignals=ptCAN_AMK_Setpoints1_Right,ptCAN_AMK_Setpoints1_Left
  Constant : Constant
  Constant1 : Constant  Value=0
  Constant2 : Constant
  Constant3 : Constant  Value=0
  Manual Switch : ManualSwitch  CurrentSetting=0
  Manual Switch1 : ManualSwitch
  pt_CAN_OUT : Outport
  wires:
  pt_CAN_IN/1 -> Bus Selector/1
  Bus Selector/2 -> AMK_PLANT/2(ptCAN_AMK1_Setpoints1)  "<ptCAN_AMK_Setpoints1_Left>"
  Bus Selector/1 -> AMK_PLANT/1(ptCAN_AMK0_Setpoints1)  "<ptCAN_AMK_Setpoints1_Right>"
  Manual Switch/1 -> AMK_PLANT/3(X140)
  Constant/1 -> Manual Switch/1
  Constant1/1 -> Manual Switch/2
  Constant2/1 -> Manual Switch1/1
  Constant3/1 -> Manual Switch1/2
  Manual Switch1/1 -> AMK_PLANT/4(LV_Enable)
  AMK_PLANT/1(ptCAN_AMK0_ActualValues1) -> Bus Creator/1  "ptCAN_AMK0_ActualValues1"
  AMK_PLANT/2(ptCAN_AMK0_ActualValues2) -> Bus Creator/2  "ptCAN_AMK0_ActualValues2"
  Bus Creator/1 -> pt_CAN_OUT/1
  AMK_PLANT/3(ptCAN_AMK1_ActualValues1) -> Bus Creator/3  "ptCAN_AMK1_ActualValues1"
  AMK_PLANT/4(ptCAN_AMK1_ActualValues2) -> Bus Creator/4  "ptCAN_AMK1_ActualValues2"

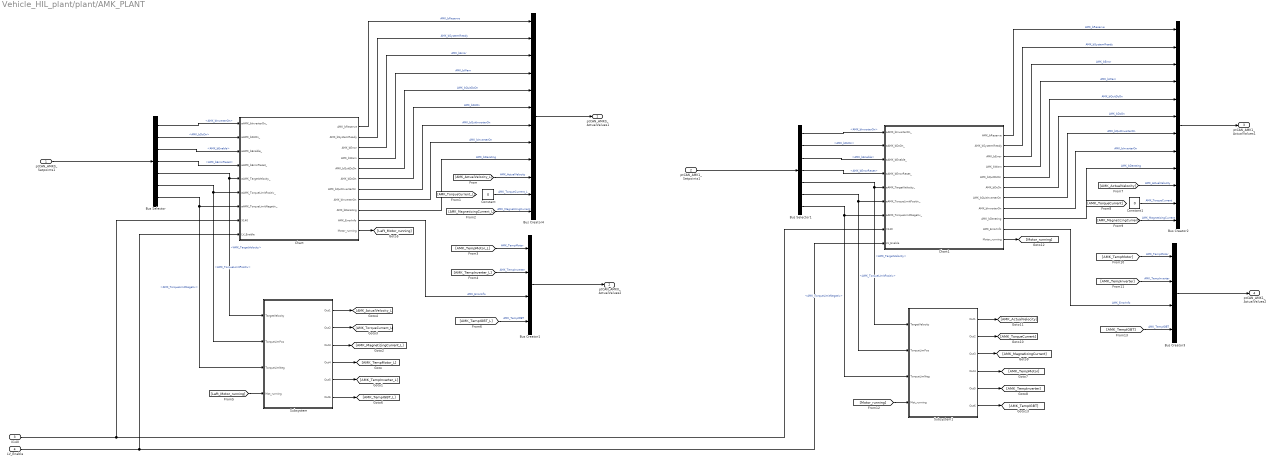
== system Vehicle_HIL_plant/plant/AMK_PLANT ==
  ptCAN_AMK0_Setpoints1 : Inport
  ptCAN_AMK1_Setpoints1 : Inport  Port=2
  X140 : Inport  Port=3
  LV_Enable : Inport  Port=4
  Bus Creator1 : BusCreator  Inputs=4
  Bus Creator2 : BusCreator  Inputs=12
  Bus Creator3 : BusCreator  Inputs=4
  Bus Creator4 : BusCreator  Inputs=12
  Bus Selector : BusSelector  OutputSignals=AMK_bInverterOn,AMK_bDcOn,AMK_bEnable,AMK_bErrorReset,AMK_TargetVelocity,AMK_TorqueLimitPositiv,AMK_TorqueLimitNegativ
  Bus Selector1 : BusSelector  OutputSignals=AMK_bInverterOn,AMK_bDcOn,AMK_bEnable,AMK_bErrorReset,AMK_TargetVelocity,AMK_TorqueLimitPositiv,AMK_TorqueLimitNegativ
  Chart : Stateflow chart  TreatAsAtomicUnit=on
  Chart1 : Stateflow chart  TreatAsAtomicUnit=on
  Constant : Constant  Value=0
  Constant1 : Constant  Value=0
  Subsystem : Subsystem
  Subsystem1 : Subsystem
  ptCAN_AMK0_ActualValues1 : Outport
  ptCAN_AMK0_ActualValues2 : Outport  Port=2
  ptCAN_AMK1_ActualValues1 : Outport  Port=3
  ptCAN_AMK1_ActualValues2 : Outport  Port=4
  wires:
  Subsystem/6(Out6) -> [AMK_TempIGBT_L]
  Subsystem/1(Out1) -> [AMK_ActualVelocity_L]
  Subsystem/2(Out2) -> [AMK_TorqueCurrent_L]
  Subsystem/3(Out3) -> [AMK_MagnetizingCurrent_L]
  Subsystem/4(Out4) -> [AMK_TempMotor_L]
  Subsystem/5(Out5) -> [AMK_TempInverter_L]
  [Left_Motor_running] -> Subsystem/4(Mot_running)
  Chart/11(Motor_running) -> [Left_Motor_running]
  Bus Selector/7 -> Subsystem/3(TorqueLimNeg), Chart/7(aAMK_TorqueLimitNegativ_)  "<AMK_TorqueLimitNegativ>"
  Bus Selector/6 -> Subsystem/2(TorqueLimPos), Chart/6(aAMK_TorqueLimitPositiv_)  "<AMK_TorqueLimitPositiv>"
  Bus Selector/5 -> Subsystem/1(TargetVelocity), Chart/5(aAMK_TargetVelocity_)  "<AMK_TargetVelocity>"
  Bus Selector/4 -> Chart/4(aAMK_bErrorReset_)  "<AMK_bErrorReset>"
  Bus Selector/3 -> Chart/3(aAMK_bEnable_)  "<AMK_bEnable>"
  Bus Selector/2 -> Chart/2(aAMK_bDcOn_)  "<AMK_bDcOn>"
  Bus Selector/1 -> Chart/1(aAMK_bInverterOn_)  "<AMK_bInverterOn>"
  ptCAN_AMK0_Setpoints1/1 -> Bus Selector/1
  Bus Creator1/1 -> ptCAN_AMK0_ActualValues2/1
  [AMK_TempMotor_L] -> Bus Creator1/1  "AMK_TempMotor"
  [AMK_TempIGBT_L] -> Bus Creator1/4  "AMK_TempIGBT"
  [AMK_TempInverter_L] -> Bus Creator1/2  "AMK_TempInverter"
  Chart/10(AMK_ErrorInfo) -> Bus Creator1/3  "AMK_ErrorInfo"
  LV_Enable/1 -> Chart1/9(LV_Enable), Chart/9(LV_Enable)
  Chart1/7(AMK_bQuitInverterOn) -> Bus Creator2/7  "AMK_bQuitInverterOn"
  [Motor_running] -> Subsystem1/4(Mot_running)
  X140/1 -> Chart/8(X140), Chart1/8(X140)
  Chart1/4(AMK_bWarn) -> Bus Creator2/4  "AMK_bWarn"
  Bus Creator2/1 -> ptCAN_AMK1_ActualValues1/1
  Chart1/10(AMK_ErrorInfo) -> Bus Creator3/3  "AMK_ErrorInfo"
  Chart1/6(AMK_bDcOn) -> Bus Creator2/6  "AMK_bDcOn"
  Chart1/1(AMK_bReserve) -> Bus Creator2/1  "AMK_bReserve"
  [AMK_TempInverter] -> Bus Creator3/2  "AMK_TempInverter"
  Bus Selector1/7 -> Subsystem1/3(TorqueLimNeg), Chart1/7(aAMK_TorqueLimitNegativ_)  "<AMK_TorqueLimitNegativ>"
  Chart1/3(AMK_bError) -> Bus Creator2/3  "AMK_bError"
  Chart1/9(AMK_bDerating) -> Bus Creator2/9  "AMK_bDerating"
  ptCAN_AMK1_Setpoints1/1 -> Bus Selector1/1
  Bus Selector1/4 -> Chart1/4(aAMK_bErrorReset_)  "<AMK_bErrorReset>"
  Bus Selector1/2 -> Chart1/2(aAMK_bDcOn_)  "<AMK_bDcOn>"
  [AMK_TempIGBT] -> Bus Creator3/4  "AMK_TempIGBT"
  Chart1/5(AMK_bQuitDcOn) -> Bus Creator2/5  "AMK_bQuitDcOn"
  Bus Selector1/1 -> Chart1/1(aAMK_bInverterOn_)  "<AMK_bInverterOn>"
  Subsystem1/3(Out3) -> [AMK_MagnetizingCurrent]
  Chart1/2(AMK_bSystemReady) -> Bus Creator2/2  "AMK_bSystemReady"
  Bus Selector1/5 -> Subsystem1/1(TargetVelocity), Chart1/5(aAMK_TargetVelocity_)  "<AMK_TargetVelocity>"
  [AMK_TempMotor] -> Bus Creator3/1  "AMK_TempMotor"
  Subsystem1/1(Out1) -> [AMK_ActualVelocity]
  Chart1/8(AMK_bInverterOn) -> Bus Creator2/8  "AMK_bInverterOn"
  Subsystem1/2(Out2) -> [AMK_TorqueCurrent]
  Subsystem1/6(Out6) -> [AMK_TempIGBT]
  Bus Selector1/3 -> Chart1/3(aAMK_bEnable_)  "<AMK_bEnable>"
  Subsystem1/5(Out5) -> [AMK_TempInverter]
  Chart1/11(Motor_running) -> [Motor_running]
  [AMK_ActualVelocity] -> Bus Creator2/10  "AMK_ActualVelocity"
  Subsystem1/4(Out4) -> [AMK_TempMotor]
  Bus Selector1/6 -> Subsystem1/2(TorqueLimPos), Chart1/6(aAMK_TorqueLimitPositiv_)  "<AMK_TorqueLimitPositiv>"
  Bus Creator3/1 -> ptCAN_AMK1_ActualValues2/1
  [AMK_MagnetizingCurrent] -> Bus Creator2/12  "AMK_MagnetizingCurrent"
  Chart/7(AMK_bQuitInverterOn) -> Bus Creator4/7  "AMK_bQuitInverterOn"
  [AMK_ActualVelocity_L] -> Bus Creator4/10  "AMK_ActualVelocity"
  Chart/8(AMK_bInverterOn) -> Bus Creator4/8  "AMK_bInverterOn"
  Chart/5(AMK_bQuitDcOn) -> Bus Creator4/5  "AMK_bQuitDcOn"
  Chart/2(AMK_bSystemReady) -> Bus Creator4/2  "AMK_bSystemReady"
  Chart/4(AMK_bWarn) -> Bus Creator4/4  "AMK_bWarn"
  Chart/9(AMK_bDerating) -> Bus Creator4/9  "AMK_bDerating"
  Chart/6(AMK_bDcOn) -> Bus Creator4/6  "AMK_bDcOn"
  Chart/3(AMK_bError) -> Bus Creator4/3  "AMK_bError"
  Bus Creator4/1 -> ptCAN_AMK0_ActualValues1/1
  [AMK_MagnetizingCurrent_L] -> Bus Creator4/12  "AMK_MagnetizingCurrent"
  Chart/1(AMK_bReserve) -> Bus Creator4/1  "AMK_bReserve"
  Constant/1 -> Bus Creator4/11  "AMK_TorqueCurrent_L"
  Constant1/1 -> Bus Creator2/11  "AMK_TorqueCurrent"

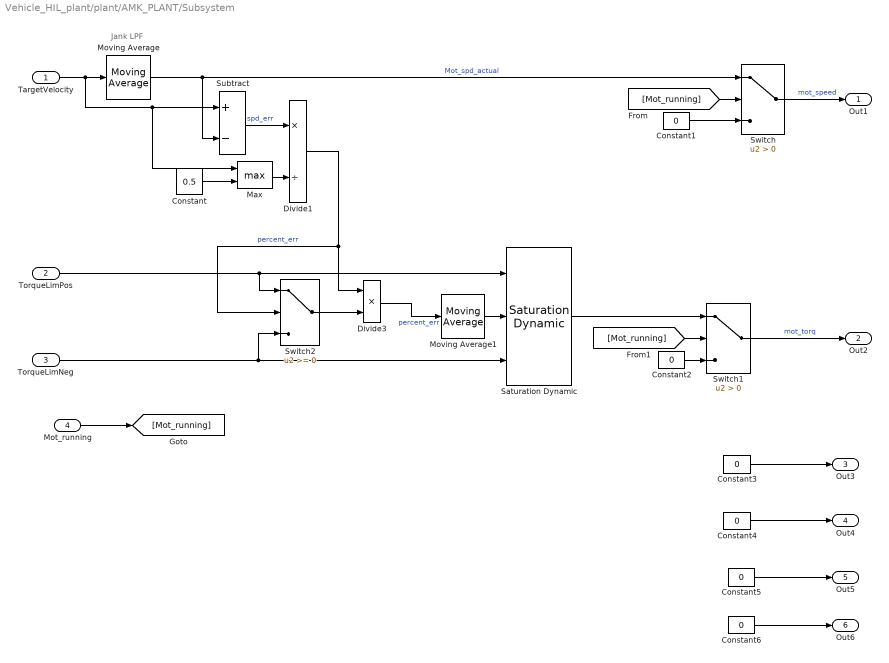
== system Vehicle_HIL_plant/plant/AMK_PLANT/Subsystem ==
  note: Jank LPF
  TargetVelocity : Inport
  TorqueLimPos : Inport  Port=2
  TorqueLimNeg : Inport  Port=3
  Mot_running : Inport  Port=4
  Constant : Constant  Value=0.5
  Constant1 : Constant  Value=0
  Constant2 : Constant  Value=0
  Constant{3..6} (4 alike) : Constant  Value=0  OutDataTypeStr=single
  Divide1 : Product  Inputs=*/
  Divide3 : Product  Inputs=**
  Max : MinMax  Function=max  Inputs=2
  Moving Average : dspstat3/Moving Average  Method=Sliding window  ForgettingFactorPort=off  SpecifyWindowLength=on  WindowLength=10  OverlapLength=9  AllowArbitraryInputLength=off  ForgettingFactor=0.9  SimulateUsing=Code generation
  Moving Average1 : dspstat3/Moving Average  Method=Sliding window  ForgettingFactorPort=off  SpecifyWindowLength=on  WindowLength=3  OverlapLength=2  AllowArbitraryInputLength=off  ForgettingFactor=0.9  SimulateUsing=Code generation
  Saturation Dynamic : simulink/Discontinuities/Saturation Dynamic  OutMin=[]  OutMax=[]  OutDataTypeStr=Inherit: Same as second input  OutDataType=fixdt(1, 16)  OutScaling=2^-10  DoSatur=off
  Subtract : Sum  Inputs=+-
  Switch : Switch  Criteria=u2 > Threshold  OutDataTypeStr=single  SaturateOnIntegerOverflow=off  InputSameDT=off
  Switch1 : Switch  Criteria=u2 > Threshold  OutDataTypeStr=single  SaturateOnIntegerOverflow=off  InputSameDT=off
  Switch2 : Switch  SaturateOnIntegerOverflow=off  InputSameDT=off
  Out1 : Outport
  Out2 : Outport  Port=2
  Out3 : Outport  Port=3
  Out4 : Outport  Port=4
  Out5 : Outport  Port=5
  Out6 : Outport  Port=6
  wires:
  Max/1 -> Divide1/2
  Constant/1 -> Max/2
  Constant6/1 -> Out6/1
  Divide3/1 -> Moving Average1/1  "percent_err"
  Moving Average1/1 -> Saturation Dynamic/2
  TorqueLimNeg/1 -> Saturation Dynamic/3, Switch2/3
  Switch2/1 -> Divide3/2
  TorqueLimPos/1 -> Switch2/1, Saturation Dynamic/1
  Constant5/1 -> Out5/1
  Constant4/1 -> Out4/1
  Constant3/1 -> Out3/1
  Divide1/1 -> Switch2/2, Divide3/1  "percent_err"
  TargetVelocity/1 -> Moving Average/1, Subtract/1, Max/1
  Subtract/1 -> Divide1/1  "spd_err"
  Switch1/1 -> Out2/1  "mot_torq"
  Saturation Dynamic/1 -> Switch1/1
  [Mot_running] -> Switch1/2
  Constant2/1 -> Switch1/3
  Moving Average/1 -> Subtract/2, Switch/1  "Mot_spd_actual"
  Constant1/1 -> Switch/3
  Switch/1 -> Out1/1  "mot_speed"
  [Mot_running] -> Switch/2
  Mot_running/1 -> [Mot_running]

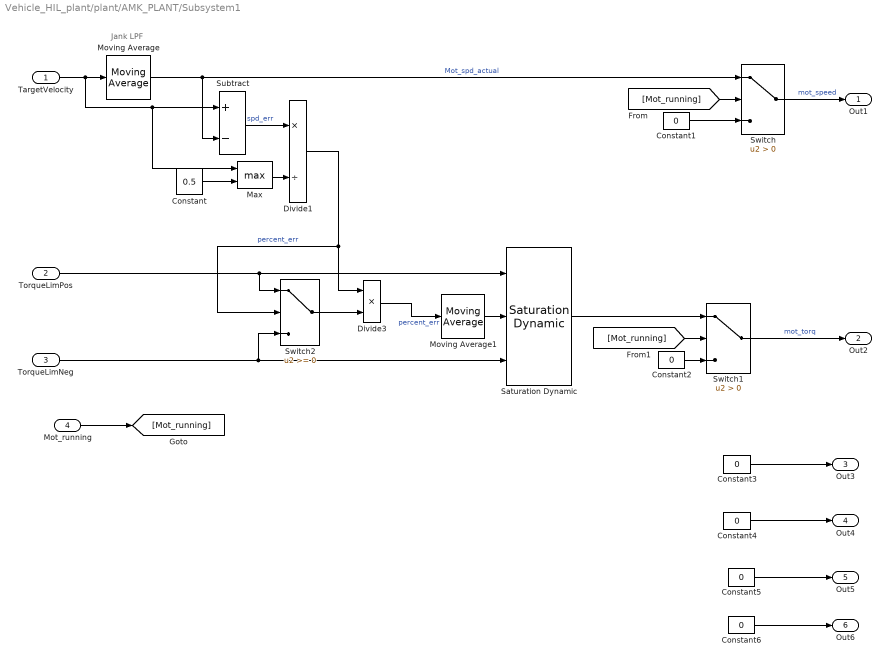
== system Vehicle_HIL_plant/plant/AMK_PLANT/Subsystem1 ==
  note: Jank LPF
  TargetVelocity : Inport
  TorqueLimPos : Inport  Port=2
  TorqueLimNeg : Inport  Port=3
  Mot_running : Inport  Port=4
  Constant : Constant  Value=0.5
  Constant1 : Constant  Value=0
  Constant2 : Constant  Value=0
  Constant{3..6} (4 alike) : Constant  Value=0  OutDataTypeStr=single
  Divide1 : Product  Inputs=*/
  Divide3 : Product  Inputs=**
  Max : MinMax  Function=max  Inputs=2
  Moving Average : dspstat3/Moving Average  Method=Sliding window  ForgettingFactorPort=off  SpecifyWindowLength=on  WindowLength=10  OverlapLength=9  AllowArbitraryInputLength=off  ForgettingFactor=0.9  SimulateUsing=Code generation
  Moving Average1 : dspstat3/Moving Average  Method=Sliding window  ForgettingFactorPort=off  SpecifyWindowLength=on  WindowLength=3  OverlapLength=2  AllowArbitraryInputLength=off  ForgettingFactor=0.9  SimulateUsing=Code generation
  Saturation Dynamic : simulink/Discontinuities/Saturation Dynamic  OutMin=[]  OutMax=[]  OutDataTypeStr=Inherit: Same as second input  OutDataType=fixdt(1, 16)  OutScaling=2^-10  DoSatur=off
  Subtract : Sum  Inputs=+-
  Switch : Switch  Criteria=u2 > Threshold  OutDataTypeStr=single  SaturateOnIntegerOverflow=off  InputSameDT=off
  Switch1 : Switch  Criteria=u2 > Threshold  OutDataTypeStr=single  SaturateOnIntegerOverflow=off  InputSameDT=off
  Switch2 : Switch  SaturateOnIntegerOverflow=off  InputSameDT=off
  Out1 : Outport
  Out2 : Outport  Port=2
  Out3 : Outport  Port=3
  Out4 : Outport  Port=4
  Out5 : Outport  Port=5
  Out6 : Outport  Port=6
  wires:
  Max/1 -> Divide1/2
  Constant/1 -> Max/2
  Constant6/1 -> Out6/1
  Divide3/1 -> Moving Average1/1  "percent_err"
  Moving Average1/1 -> Saturation Dynamic/2
  TorqueLimNeg/1 -> Saturation Dynamic/3, Switch2/3
  Switch2/1 -> Divide3/2
  TorqueLimPos/1 -> Switch2/1, Saturation Dynamic/1
  Constant5/1 -> Out5/1
  Constant4/1 -> Out4/1
  Constant3/1 -> Out3/1
  Divide1/1 -> Switch2/2, Divide3/1  "percent_err"
  TargetVelocity/1 -> Moving Average/1, Subtract/1, Max/1
  Subtract/1 -> Divide1/1  "spd_err"
  Switch1/1 -> Out2/1  "mot_torq"
  Saturation Dynamic/1 -> Switch1/1
  [Mot_running] -> Switch1/2
  Constant2/1 -> Switch1/3
  Moving Average/1 -> Subtract/2, Switch/1  "Mot_spd_actual"
  Constant1/1 -> Switch/3
  Switch/1 -> Out1/1  "mot_speed"
  [Mot_running] -> Switch/2
  Mot_running/1 -> [Mot_running]

== stateflow chart Vehicle_HIL_plant/plant/AMK_PLANT/Chart1 ==
  state AMK_idle
    en:
    AMK_bReserve = 0;
    AMK_bSystemReady = 0;
    AMK_bError = 0;
    AMK_bWarn = 0;
    AMK_bQuitDcOn = 0;
    AMK_bDcOn = 0;
    AMK_bQuitInverterOn = 0;
    AMK_bInverterOn = 0;
    AMK_bDerating = 0;
    AMK_ErrorInfo = 0;
    Motor_running = false;
  state LV_ON
    state Enable_System_Ready
      en:
      AMK_bSystemReady = 1;
    state bQuitDcOff
      en:
      AMK_bQuitDcOn = 0
    state Enable_Quit_Dc_On
      en:
      AMK_bQuitDcOn = 1;
      AMK_bDcOn = 1;
    state bDcOff
      en:
      AMK_bDcOn = 0
    state Inverter_Stuff2
      % (*3) and %(*4)
    state Inverter
    state bEnable_off
      en:
      AMK_bQuitDcOn = 0
    state Inventer_On
      en:
      AMK_bInverterOn = 1;
    state bInverter_off
      en:
      AMK_bInverterOn = 0
    state Quit_Inventer_On
      en:
      AMK_bQuitInverterOn =1;
    state Motor_running
      en:
      Motor_running = true;
    state Shut_off_start
      en:
      AMK_bQuitInverterOn =0;
    (default) -> Enable_System_Ready
    Enable_System_Ready -> (junction 99) : [aAMK_bDcOn_ == 1]
    (junction 99) -> Enable_Quit_Dc_On : after(250,msec)
    bDcOff -> bQuitDcOff
    Enable_Quit_Dc_On -> Inverter : [(abs(aAMK_TargetVelocity_) == 0) && ...
        | (abs(aAMK_TorqueLimitPositiv_) == 0) && ...
        | (abs(aAMK_TorqueLimitNegativ_) == 0)]
    Inverter_Stuff2 -> bDcOff : [aAMK_bDcOn_ == 0]
    bEnable_off -> Inverter_Stuff2
    Inverter -> (junction 101) : [(aAMK_bEnable_ == 1) && ...
        | (aAMK_bInverterOn_ == 1)]
    (junction 101) -> Inventer_On : after(250,msec)
    bInverter_off -> bEnable_off : [aAMK_bEnable_ == 0]
    Inventer_On -> Quit_Inventer_On : [X140 == 1]
    Shut_off_start -> bInverter_off [order 2] : [aAMK_bInverterOn_ == 0]
    Shut_off_start -> Quit_Inventer_On [order 1] : [X140 == 1]
    Quit_Inventer_On -> Motor_running : after(250,msec)
    Motor_running -> Shut_off_start : [X140 == 0]
  (default) -> AMK_idle
  AMK_idle -> LV_ON : [LV_Enable == 1]
  LV_ON -> AMK_idle : [LV_Enable == 0]
  data: aAMK_bInverterOn_ input; aAMK_bDcOn_ input; aAMK_bEnable_ input; aAMK_bErrorReset_ input; aAMK_TargetVelocity_ input; aAMK_TorqueLimitPositiv_ input; aAMK_TorqueLimitNegativ_ input; AMK_bReserve output uint8; AMK_bSystemReady output uint8; AMK_bError output uint8; AMK_bWarn output uint8; AMK_bQuitDcOn output uint8; AMK_bDcOn output uint8; AMK_bQuitInverterOn output uint8; AMK_bInverterOn output uint8; AMK_bDerating output uint8; AMK_ErrorInfo output int32; Motor_running output boolean =false; X140 input; LV_Enable input

== stateflow chart Vehicle_HIL_plant/plant/AMK_PLANT/Chart ==
  state AMK_idle
    en:
    AMK_bReserve = 0;
    AMK_bSystemReady = 0;
    AMK_bError = 0;
    AMK_bWarn = 0;
    AMK_bQuitDcOn = 0;
    AMK_bDcOn = 0;
    AMK_bQuitInverterOn = 0;
    AMK_bInverterOn = 0;
    AMK_bDerating = 0;
    AMK_ErrorInfo = 0;
    Motor_running = false;
  state LV_ON
    state Enable_System_Ready
      en:
      AMK_bSystemReady = 1;
    state bQuitDcOff
      en:
      AMK_bQuitDcOn = 0
    state Enable_Quit_Dc_On
      en:
      AMK_bQuitDcOn = 1;
      AMK_bDcOn = 1;
    state bDcOff
      en:
      AMK_bDcOn = 0
    state Inverter_Stuff2
      % (*3) and %(*4)
    state Inverter
    state bEnable_off
      en:
      AMK_bQuitDcOn = 0
    state Inventer_On
      en:
      AMK_bInverterOn = 1;
    state bInverter_off
      en:
      AMK_bInverterOn = 0
    state Quit_Inventer_On
      en:
      AMK_bQuitInverterOn =1;
    state Motor_running
      en:
      Motor_running = true;
    state Shut_off_start
      en:
      AMK_bQuitInverterOn =0;
    (default) -> Enable_System_Ready
    Enable_System_Ready -> (junction 99) : [aAMK_bDcOn_ == 1]
    (junction 99) -> Enable_Quit_Dc_On : after(250,msec)
    bDcOff -> bQuitDcOff
    Enable_Quit_Dc_On -> Inverter : [(abs(aAMK_TargetVelocity_) == 0) && ...
        | (abs(aAMK_TorqueLimitPositiv_) == 0) && ...
        | (abs(aAMK_TorqueLimitNegativ_) == 0)]
    Inverter_Stuff2 -> bDcOff : [aAMK_bDcOn_ == 0]
    bEnable_off -> Inverter_Stuff2
    Inverter -> (junction 101) : [(aAMK_bEnable_ == 1) && ...
        | (aAMK_bInverterOn_ == 1)]
    (junction 101) -> Inventer_On : after(250,msec)
    bInverter_off -> bEnable_off : [aAMK_bEnable_ == 0]
    Inventer_On -> Quit_Inventer_On : [X140 == 1]
    Shut_off_start -> bInverter_off [order 2] : [aAMK_bInverterOn_ == 0]
    Shut_off_start -> Quit_Inventer_On [order 1] : [X140 == 1]
    Quit_Inventer_On -> Motor_running : after(250,msec)
    Motor_running -> Shut_off_start : [X140 == 0]
  (default) -> AMK_idle
  AMK_idle -> LV_ON : [LV_Enable == 1]
  LV_ON -> AMK_idle : [LV_Enable == 0]
  data: aAMK_bInverterOn_ input; aAMK_bDcOn_ input; aAMK_bEnable_ input; aAMK_bErrorReset_ input; aAMK_TargetVelocity_ input; aAMK_TorqueLimitPositiv_ input; aAMK_TorqueLimitNegativ_ input; AMK_bReserve output uint8; AMK_bSystemReady output uint8; AMK_bError output uint8; AMK_bWarn output uint8; AMK_bQuitDcOn output uint8; AMK_bDcOn output uint8; AMK_bQuitInverterOn output uint8; AMK_bInverterOn output uint8; AMK_bDerating output uint8; AMK_ErrorInfo output int32; Motor_running output boolean =false; X140 input; LV_Enable input
